simulink model "gen"  (R2025b)
settings: Solver=FixedStepDiscrete  StartTime=0.0  StopTime=inf  FixedStep=0.02  RelTol=1e-3
libraries: dspmathops x1
settings Model: Creator=Huawei  LastModifiedBy=lolve
settings OptimizationCC: BlockReduction=off  UseDivisionForNetSlopeComputation=on  OptimizeBlockIOStorage=off

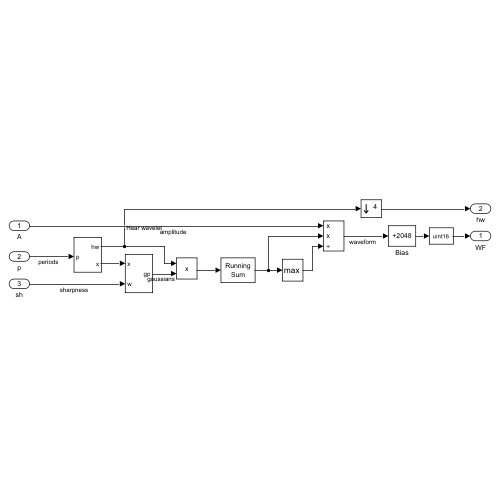
[thumbnail: Simulink's stored preview of the top-level diagram]
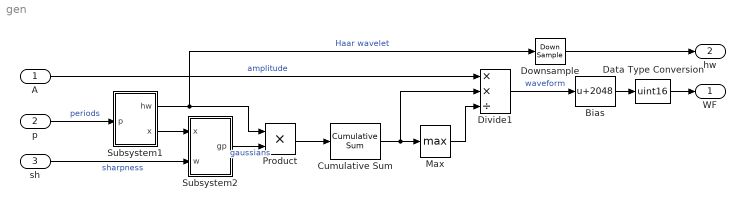
== system gen ==
  A : Inport  PortDimensions=1
  p : Inport  Port=2  PortDimensions=1
  sh : Inport  Port=3  PortDimensions=1
  Bias : Bias  Bias=2048  SaturateOnIntegerOverflow=off
  Cumulative Sum : dspmathops/Cumulative Sum  dim=Channels (running sum)  InputProcessing=Columns as channels (frame based)  reset_popup=None  roundingMode=Floor  overflowMode=off  outputDataTypeStr=Inherit: Same as accumulator  outputMin=[]  outputMax=[]  outputLastDataTypeStr=Inherit: Same as accumulator
  Data Type Conversion : DataTypeConversion  OutDataTypeStr=uint16  RndMeth=Round  SaturateOnIntegerOverflow=off
  Divide1 : Product  Inputs=**/
  Downsample : DownSample  N=4
  Max : MinMax  Function=max
  Product : Product
  Subsystem1 : Subsystem
  Subsystem2 : Subsystem
  WF : Outport
  hw : Outport  Port=2
  wires:
  Bias/1 -> Data Type Conversion/1
  A/1 -> Divide1/1  "amplitude"
  Subsystem2/1(gp) -> Product/2  "gaussians"
  Subsystem1/1(hw) -> Downsample/1, Product/1  "Haar wavelet"
  sh/1 -> Subsystem2/2(w)  "sharpness"
  Data Type Conversion/1 -> WF/1
  Max/1 -> Divide1/3
  Subsystem1/2(x) -> Subsystem2/1(x)
  Divide1/1 -> Bias/1  "waveform"
  p/1 -> Subsystem1/1(p)  "periods"
  Cumulative Sum/1 -> Divide1/2, Max/1
  Product/1 -> Cumulative Sum/1
  Downsample/1 -> hw/1

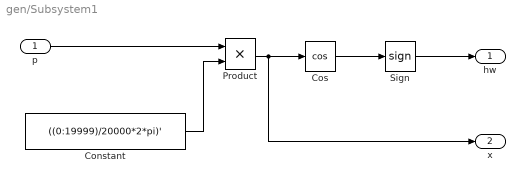
== system gen/Subsystem1 ==
  p : Inport
  Constant : Constant  Value=((0:19999)/20000*2*pi)'
  Cos : Trigonometry  Operator=cos
  Product : Product
  Sign : Signum
  hw : Outport  PortDimensions=[20000 1]
  x : Outport  Port=2  PortDimensions=[20000 1]
  wires:
  Cos/1 -> Sign/1
  Product/1 -> x/1, Cos/1
  Constant/1 -> Product/2
  p/1 -> Product/1
  Sign/1 -> hw/1

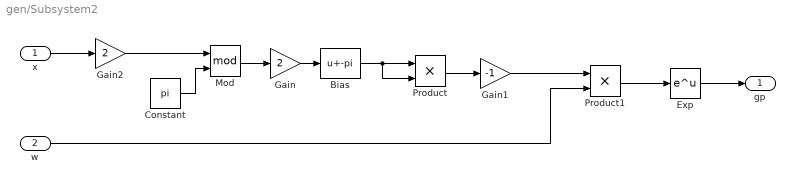
== system gen/Subsystem2 ==
  x : Inport
  w : Inport  Port=2
  Bias : Bias  Bias=-pi  SaturateOnIntegerOverflow=off
  Constant : Constant  Value=pi
  Exp : Math
  Gain : Gain  Gain=2
  Gain1 : Gain  Gain=-1
  Gain2 : Gain  Gain=2
  Mod : Math  Operator=mod
  Product : Product
  Product1 : Product
  gp : Outport
  wires:
  x/1 -> Gain2/1
  Constant/1 -> Mod/2
  Mod/1 -> Gain/1
  Gain/1 -> Bias/1
  Bias/1 -> Product/2, Product/1
  Product/1 -> Gain1/1
  Gain1/1 -> Product1/1
  Exp/1 -> gp/1
  Product1/1 -> Exp/1
  w/1 -> Product1/2
  Gain2/1 -> Mod/1
